simulink model "lab3_linear"  (R2022a)
settings: Solver=VariableStepAuto  StartTime=0.0  StopTime=30.0  RelTol=1e-10  AbsTol=1e-10
undefined symbols (not defined in the file or in its folder): A, B, K, x0
settings Model: Creator=sun  LastModifiedBy=yuans
settings ModelReferenceCC: EnableRefExpFcnMdlSchedulingChecks=off
settings RTWCC: Description=Generic Real-Time Target  GPUComputeCapability=5.0

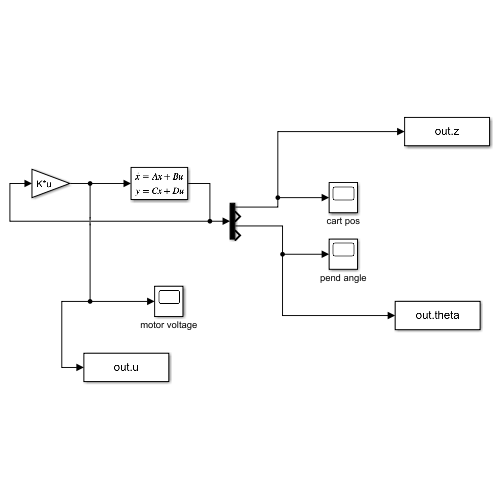
[thumbnail: Simulink's stored preview of the top-level diagram]
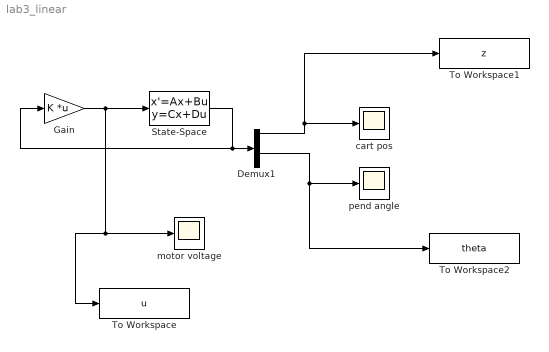
== system lab3_linear ==
  Demux1 : Demux
  Gain : Gain  Gain=K  Multiplication=Matrix(K*u)
  State-Space : StateSpace  A=A  B=B  C=eye(4)  D=zeros(4,1)  InitialCondition=x0
  To Workspace : ToWorkspace  VariableName=u  SaveFormat=Timeseries  SampleTime=-1
  To Workspace1 : ToWorkspace  VariableName=z  SaveFormat=Timeseries  SampleTime=-1
  To Workspace2 : ToWorkspace  VariableName=theta  SaveFormat=Timeseries  SampleTime=-1
  cart pos : Scope
  motor voltage : Scope
  pend angle : Scope
  wires:
  State-Space/1 -> Demux1/1, Gain/1
  Gain/1 -> To Workspace/1, motor voltage/1, State-Space/1
  Demux1/1 -> To Workspace1/1, cart pos/1
  Demux1/3 -> To Workspace2/1, pend angle/1
